simulink model "PLL_type2_noise"  (R2014b)
settings: Solver=VariableStepDiscrete  StartTime=0.0  StopTime=(n-1)*T  RelTol=1e-3
PreLoadFcn:
  | %%%%%%%%%%%%%%%%%%%%%%%%%%%%%%%%%%%%%%%%%%%%%%%%%%%%%%%%%%%%%%%%%%%%%%%%%%%
  | % check to see if Simulink library folder is missing from the MATLAB path %
  | %%%%%%%%%%%%%%%%%%%%%%%%%%%%%%%%%%%%%%%%%%%%%%%%%%%%%%%%%%%%%%%%%%%%%%%%%%%
  | if isempty(strfind(path, 'rtlsdr_book_library'))
  | 
  |     % create error window
  |     fig_error = figure(...
  |         'Name', 'Error: RTL-SDR Book Library',...
  |         'Toolbar','none',...
  |         'MenuBar','none',...
  |         'NumberTitle','off',...
  |         'Resize','off',...
  |         'WindowStyle','modal');
  |     fig_error.Position(3) = 600;
  |     fig_error.Position(4) = 150;
  |     fig_axes = axes(...
  |         'Parent',fig_error,...
  |         'Position',[0,0,1,1],...
  |         'visible','off');
  |     % error message
  |     t_title = text(.05,.8,...
  |         'MISSING DIRECTORIES',...
  |         'FontSize',11.5);
  |     t_body = text(.075,.6,...
  |         [{'Simulink cannot find the  \it{<root>}\rm / \it{rtlsdr\_book\_library}\rm  folder in the \it{MATLAB Path}\rm.'},...
  |         {'Please set the MATLAB path following the instructions given in Exercise 2.4.'}],...
  |         'FontSize',10.5);
  |     % buttons
  |     btn_path = uicontrol(...
  |         'Parent',fig_error,...
  |         'String','Set Path Now',...
  |         'FontSize',10,...
  |         'Callback', 'pathtool; close(fig_error);',...
  |         'Position', [fig_error.Position(3)/2-210, 30, 200, 30]);
  |     btn_abort = uicontrol(...
  |         'Parent',fig_error,...
  |         'String','No thanks',...
  |         'FontSize',10,...
  |         'Callback', 'close(fig_error); abort=1;',...
  |         'Position', [fig_error.Position(3)/2+10, 30, 200, 30]);
  | 
  |     % pause to allow user to interact with error box
  |     uiwait(fig_error);
  | 
  |     % abort simulation
  |     try
  |         if abort==1
  |             set_param(gcs, 'SimulationCommand', 'stop');
  |         end
  |     end
  | 
  |     % if user has set path, allow diagram to be updated
  |     if ~exist('abort','var')
  |         % create error window
  |         fig_update = figure(...
  |             'Name', 'Update Diagram',...
  |             'Toolbar','none',...
  |             'MenuBar','none',...
  |             'NumberTitle','off',...
  |             'Resize','off');
  |         fig_update.Position(3) = 400;
  |         fig_update.Position(4) = 120;
  |         fig_axes = axes(...
  |             'Parent',fig_update,...
  |             'Position',[0,0,1,1],...
  |             'visible','off');
  |         % instruction message
  |         t_body = text(.075,.7,...
  |             'Once you have set the path, update the block diagram',...
  |             'FontSize',10.5);
  |         % button
  |         btn_update = uicontrol(...
  |             'Parent',fig_update,...
  |             'String','Update Block Diagram',...
  |             'FontSize',10,...
  |             'Callback', 'set_param(gcs,''SimulationCommand'',''update''); close(gcf)',...
  |             'Position', [fig_update.Position(3)/2-100, 30, 200, 30]);
  |     end
  | 
  |     % clear error components
  |     clear('fig_error','fig_update','fig_axes','t_title','t_body','btn_path','btn_abort','btn_update','abort');
  | 
  | end
  | %%%%%%%%%%%%%%%%%%%%%%%%%%%%%%%%%%%%%%%%%%%%%%%%%%%%%%%%%%%%%%%%%%%%%%%%%%%
  | 
  | MHz = fs/1e6;
StartFcn:
  | close all;
StopFcn:
  | doFFTplot(fs, Reference(round(length(Reference)*0.5):end), 'Reference', 1, 8, 'hann');
  | set(8,'Name','FFT Plot of Input Sine Wave (Final 50% of Simulation Time)','NumberTitle','off');
  | setStandardFigSize(8);
  | 
  | doFFTplot(fs, Synthesised(round(length(Synthesised)*0.5):end), 'Synthesised', 1, 9, 'hann');
  | set(9,'Name','FFT Plot of Synthesised Sine Wave (Final 50% of Simulation Time)','NumberTitle','off');
  | setStandardFigSize(9);
values from neighbouring files (symbols this model uses):
  awgn = 0.05    [configure_noise_model.m]
  ferr = 4500    [configure_noise_model.m]
  fq = 1e6    (= 1000000)    [configure_noise_model.m]
  fs = 10e6    (= 10000000)    [configure_noise_model.m]
  K1 = (4*d*eta)/(Ko*Kp*(1+(2*d*eta)+eta^2))    (= 0.00532515593619)    [configure_noise_model.m]
  K2 = (4*eta^2)/(Ko*Kp*(1+(2*d*eta)+eta^2))    (= 7.10092274115e-06)    [configure_noise_model.m]
  Ko = 1    [configure_noise_model.m]
undefined symbols (not defined in the file or in its folder): startfcn_time_scope
libraries: rtlsdr_book_library x1
CloseFcn:
  | closefcn_model;
Description:
  | Software, Simulation Examples and Design Exercises Licence Agreement
  | 
  | This license agreement refers to the simulation examples, design exercises and files,
  | and associated software MATLAB and Simulink resources that accompany the book:
  | 
  |      Title: Software Defined Radio using MATLAB & Simulink and the RTL-SDR
  |      Published by Strathclyde Academic Media, 2015
  |      Authored by Robert W. Stewart, Kenneth W. Barlee, Dale S.W. Atkinson,
  |      and Louise H. Crockett
  | 
  | and made available as a download from, www.desktopSDR.com or variously acquired
  | by other means such as via USB storage, cloud storage, disk or any other electronic
  | or optical or magnetic storage mechanism. These files and associated software may
  | be used subject to the terms of agreement of the conditions below:
  | 
  |     Copyright © 2015 Robert W. Stewart, Kenneth W. Barlee, Dale S.W. Atkinson,
  |     and Louise H. Crockett
  |     All rights reserved.
  | 
  | Redistribution and use in source and binary forms, with or without modification, are
  | permitted provided that the following conditions are met:
  | 
  |    1.  Redistributions of source code must retain the above copyright notice, this list of
  |         conditions and the following disclaimer.
  | 
  |    2.  Redistributions in binary form must reproduce the above copyright notice, this
  |         list of conditions and the following disclaimer in the documentation and/or other
  |         materials provided with the distribution.
  | 
  |    3.  Neither the name of the copyright holder nor the names of its contributors may
  |         be used to endorse or promote products derived from this software without
  |         specific prior written permission.
  | 
  |    4.  In all cases, the software is, and all modifications and derivatives of the
  |         software shall be, licensed to you solely for use in conjunction with The
  |         MathWorks, Inc. products and service offerings.
  | 
  | THIS SOFTWARE IS PROVIDED BY THE COPYRIGHT HOLDERS AND CONTRIBUTORS
  | "AS IS" AND ANY EXPRESS OR IMPLIED WARRANTIES, INCLUDING, BUT NOT LIMITED
  | TO, THE IMPLIED WARRANTIES OF MERCHANTABILITY AND FITNESS FOR A
  | PARTICULAR PURPOSE ARE DISCLAIMED. IN NO EVENT SHALL THE COPYRIGHT
  | HOLDER OR CONTRIBUTORS BE LIABLE FOR ANY DIRECT, INDIRECT, INCIDENTAL,
  | SPECIAL, EXEMPLARY, OR CONSEQUENTIAL DAMAGES (INCLUDING, BUT NOT
  | LIMITED TO, PROCUREMENT OF SUBSTITUTE GOODS OR SERVICES; LOSS OF USE,
  | DATA, OR PROFITS; OR BUSINESS INTERRUPTION) HOWEVER CAUSED AND ON ANY
  | THEORY OF LIABILITY, WHETHER IN CONTRACT, STRICT LIABILITY, OR TORT
  | (INCLUDING NEGLIGENCE OR OTHERWISE) ARISING IN ANY WAY OUT OF THE USE
  | OF THIS SOFTWARE, EVEN IF ADVISED OF THE POSSIBILITY OF SUCH DAMAGE.
  | 
  | 
  | Audio Tracks used in Simulations Examples and Design Exercises
  | 
  | The music and vocal files used within the Examples files and software within the book
  | were variously written, arranged, performed, recorded and produced by Garrey Rice,
  | Adam Struth, Jamie Struth, Iain Thistlethwaite and also Marshall Craigmyle who
  | collectively, and individually where appropriate, assert and retain all of their copyright,
  | performance and artistic rights. Permission to use and reproduce this music is
  | granted for all purposes associated with MATLAB and Simulink software and the
  | simulation examples and design exercises files that accompany this book. Requests to
  | use the music for any other purpose should be directed to: info@desktopSDR.com.
  | For information on music track names, full credits, and links to the musicians please
  | refer to www.desktopSDR.com/more/audio.
settings Model: Creator=desktopSDR Team  LastModifiedBy=desktopSDR Team
settings DataIOCC: LimitDataPoints=off  SaveOutput=off  SignalLogging=off  SaveTime=off
settings DebuggingCC: UnderspecifiedInitializationDetection=Classic  MergeDetectMultiDrivingBlocksExec=none

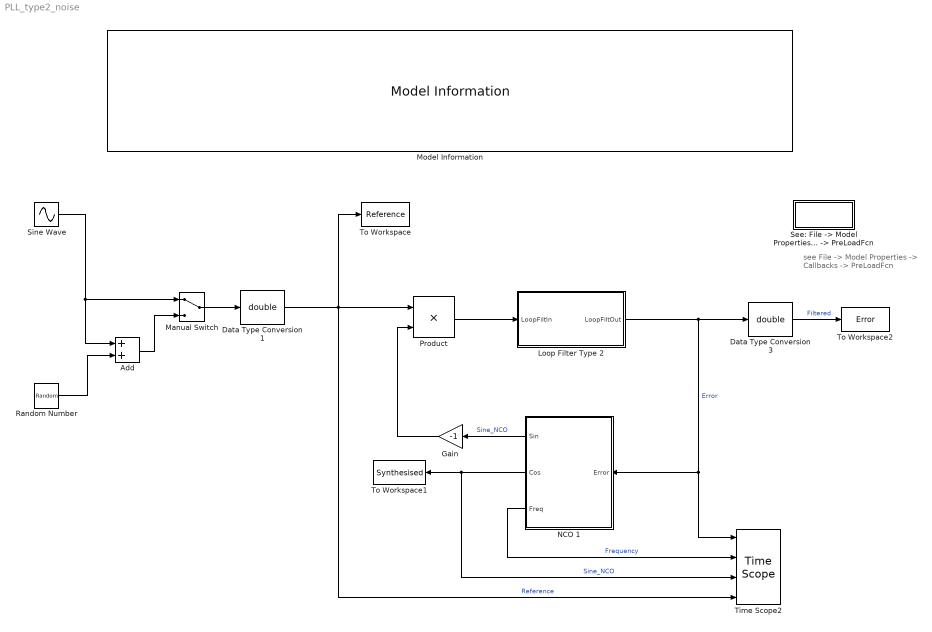
== system PLL_type2_noise ==
  note: see File -> Model Properties
      | -> Callbacks -> PreLoadFcn
  Add : Sum
  Data Type Conversion1 : DataTypeConversion  OutDataTypeStr=double  SampleTime=1/fs
  Data Type Conversion3 : DataTypeConversion  OutDataTypeStr=double  SampleTime=1/fs
  Gain : Gain  Gain=-1
  Loop Filter Type 2 : Subsystem  mask(Loop Filter (Type 2)){K1=K1, K2=K2}
      mask prompts: K1 "K1 (proportional path)"; K2 "K2 (integral path)"
      mask help: This loop filter contains two paths: a proportional path with scaling coefficient K1, and an integral path with scaling coefficient K2.
  Manual Switch : ManualSwitch
  Model Information : rtlsdr_book_library/Additional Tools/Model Information/Model Information
  NCO 1 : Subsystem
  Product : Product
  Random Number : RandomNumber  Variance=awgn  SampleTime=1/fs
  "See: File -> Model Properties -> Callbacks -> PreLoadFcn " : Subsystem
      mask Display:
      | MHz = evalin('base', 'MHz');
      | fprintf(['fs = ',num2str(MHz),' MHz']);
  Sine Wave : Sin  Frequency=2*pi*(fq+ferr)  Phase=pi/5  SampleTime=0
  Time Scope2 : TimeScope  StartFcn=startfcn_time_scope;  DefaultConfigurationName=spbscopes.TimeScopeBlockCfg  NumInputPorts=4
  To Workspace : ToWorkspace  VariableName=Reference  SampleTime=-1
  To Workspace1 : ToWorkspace  VariableName=Synthesised  SampleTime=-1
  To Workspace2 : ToWorkspace  VariableName=Error  SampleTime=-1
  wires:
  Data Type Conversion1/1 -> Time Scope2/4, Product/1, To Workspace/1  "Reference"
  Data Type Conversion3/1 -> To Workspace2/1  "Filtered"
  Loop Filter Type 2/1(LoopFiltOut) -> Time Scope2/1, NCO 1/1(Error), Data Type Conversion3/1  "Error"
  Sine Wave/1 -> Add/1, Manual Switch/1
  Manual Switch/1 -> Data Type Conversion1/1
  NCO 1/2(Cos) -> To Workspace1/1, Time Scope2/3  "Sine_NCO"
  Product/1 -> Loop Filter Type 2/1(LoopFiltIn)
  Add/1 -> Manual Switch/2
  Random Number/1 -> Add/2
  NCO 1/3(Freq) -> Time Scope2/2  "Frequency"
  NCO 1/1(Sin) -> Gain/1  "Sine_NCO"
  Gain/1 -> Product/2

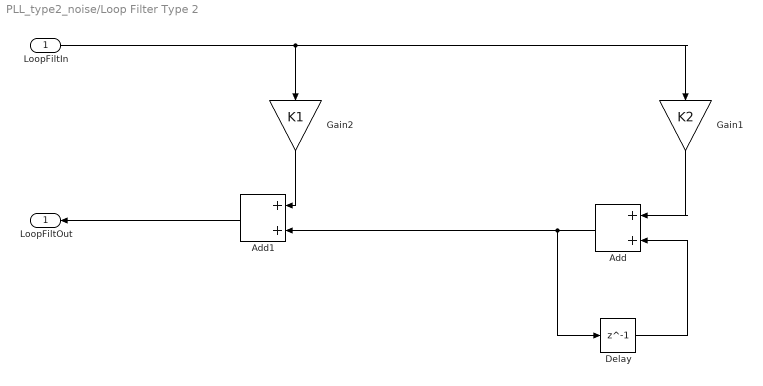
== system PLL_type2_noise/Loop Filter Type 2 ==
  LoopFiltIn : Inport
  Add : Sum
  Add1 : Sum
  Delay : Delay  DelayLength=1
  Gain1 : Gain  Gain=K2
  Gain2 : Gain  Gain=K1
  LoopFiltOut : Outport
  wires:
  Add1/1 -> LoopFiltOut/1
  Delay/1 -> Add/2
  Add/1 -> Delay/1, Add1/2
  LoopFiltIn/1 -> Gain2/1, Gain1/1
  Gain2/1 -> Add1/1
  Gain1/1 -> Add/1

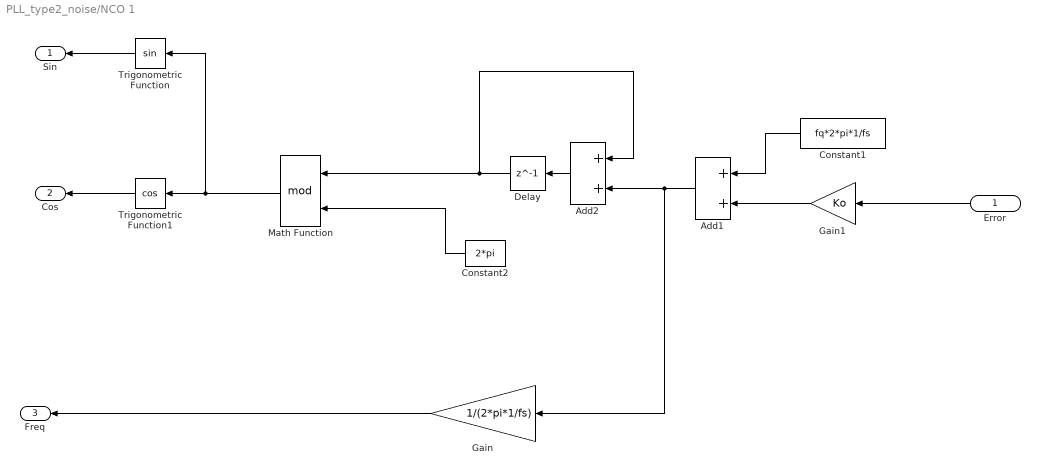
== system PLL_type2_noise/NCO 1 ==
  Error : Inport
  Add1 : Sum  AccumDataTypeStr=single
  Add2 : Sum  AccumDataTypeStr=single
  Constant1 : Constant  Value=fq*2*pi*1/fs  OutDataTypeStr=double
  Constant2 : Constant  Value=2*pi  OutDataTypeStr=double
  Delay : Delay  DelayLength=1  InitialCondition=0.001
  Gain : Gain  Gain=1/(2*pi*1/fs)
  Gain1 : Gain  Gain=Ko  OutDataTypeStr=single
  Math Function : Math  Operator=mod  SaturateOnIntegerOverflow=on
  Trigonometric Function : Trigonometry
  Trigonometric Function1 : Trigonometry  Operator=cos
  Sin : Outport
  Cos : Outport  Port=2
  Freq : Outport  Port=3
  wires:
  Gain/1 -> Freq/1
  Constant1/1 -> Add1/1
  Error/1 -> Gain1/1
  Add1/1 -> Gain/1, Add2/2
  Add2/1 -> Delay/1
  Constant2/1 -> Math Function/2
  Trigonometric Function/1 -> Sin/1
  Math Function/1 -> Trigonometric Function/1, Trigonometric Function1/1
  Trigonometric Function1/1 -> Cos/1
  Gain1/1 -> Add1/2
  Delay/1 -> Add2/1, Math Function/1

== system PLL_type2_noise/See: File -> Model Properties -> Callbacks -> PreLoadFcn  ==
